simulink model "Subsitema_mecanico_completo"  (R2021a)
settings: Solver=VariableStepAuto  StartTime=0.0  StopTime=10.0  RelTol=1e-3
undefined symbols (not defined in the file): beq, Jeq, r
settings Model: Creator=fhlla  LastModifiedBy=fhlla

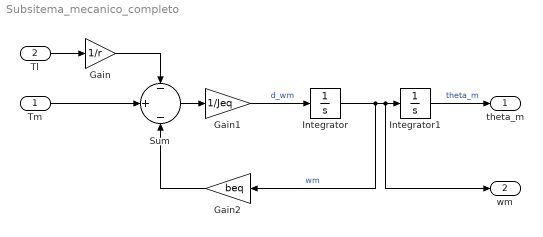
== system Subsitema_mecanico_completo ==
  Tm : Inport
  Tl : Inport  Port=2
  Gain : Gain  Gain=1/r
  Gain1 : Gain  Gain=1/Jeq
  Gain2 : Gain  Gain=beq
  Integrator : Integrator
  Integrator1 : Integrator
  Sum : Sum  Inputs=-|+|-
  theta_m : Outport
  wm : Outport  Port=2
  wires:
  Tl/1 -> Gain/1
  Gain/1 -> Sum/1
  Tm/1 -> Sum/2
  Sum/1 -> Gain1/1
  Integrator/1 -> Gain2/1, wm/1, Integrator1/1  "wm"
  Gain1/1 -> Integrator/1  "d_wm"
  Integrator1/1 -> theta_m/1  "theta_m"
  Gain2/1 -> Sum/3
